simulink model "HybridReactorController"  (R2013a)
settings: Solver=ode45  StartTime=0.0  StopTime=500  RelTol=1e-3
undefined symbols (not defined in the file or in its folder): DiscIntNeverNeededParam
settings Model: Creator=Avisek Naug  LastModifiedBy=Avisek Naug

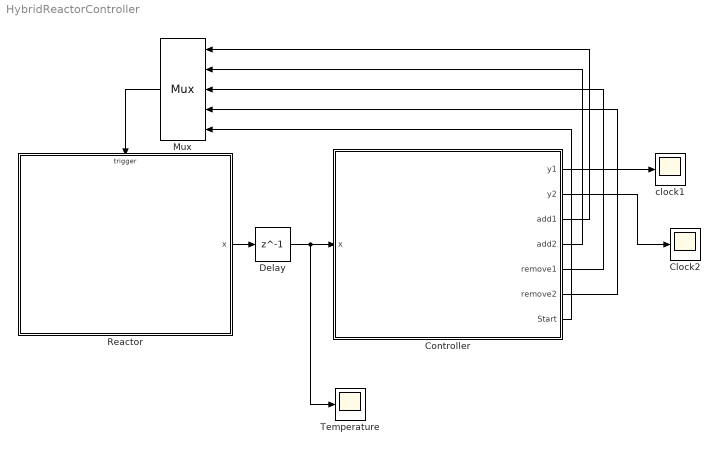
== system HybridReactorController ==
  Clock2 : Scope
      settings: SaveName=ScopeData2
  Controller : Stateflow chart  TreatAsAtomicUnit=on
  Delay : Delay  DelayLength=1  InitialCondition=0  SampleTime=5
  Mux : Mux  Inputs=5
      settings: DisplayOption=signals
  Reactor : Stateflow chart  TreatAsAtomicUnit=on
  Temperature : Scope
  clock1 : Scope
  wires:
  Reactor/1(x) -> Delay/1
  Mux/1 -> Reactor/Trigger
  Controller/3(add1) -> Mux/1
  Controller/4(add2) -> Mux/2
  Controller/5(remove1) -> Mux/3
  Controller/6(remove2) -> Mux/4
  Delay/1 -> Controller/1(x), Temperature/1
  Controller/1(y1) -> clock1/1
  Controller/2(y2) -> Clock2/1
  Controller/7(Start) -> Mux/5

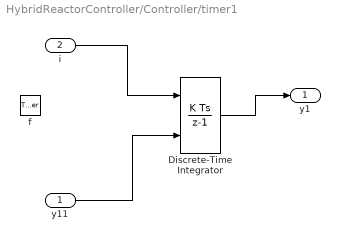
== system HybridReactorController/Controller/timer1 ==
  y11 : Inport  OutDataTypeStr=double
  i : Inport  Port=2
  f : TriggerPort  TriggerType=function-call
      settings: CopyFcn=Stateflow.SLINSF.SimulinkMan.removeBlockPreDeleteFcn  PreDeleteFcn=Stateflow.SLINSF.SimulinkMan.unsafePredeleteFcn
  Discrete-Time Integrator : DiscreteIntegrator  InitialConditionSource=external  SampleTime=-1  ICPrevOutput=DiscIntNeverNeededParam  ICPrevScaledInput=DiscIntNeverNeededParam
  y1 : Outport
  wires:
  Discrete-Time Integrator/1 -> y1/1
  i/1 -> Discrete-Time Integrator/1
  y11/1 -> Discrete-Time Integrator/2

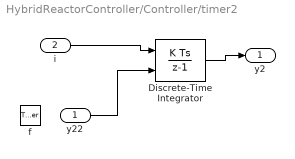
== system HybridReactorController/Controller/timer2 ==
  y22 : Inport
  i : Inport  Port=2
  f : TriggerPort  TriggerType=function-call
      settings: CopyFcn=Stateflow.SLINSF.SimulinkMan.removeBlockPreDeleteFcn  PreDeleteFcn=Stateflow.SLINSF.SimulinkMan.unsafePredeleteFcn
  Discrete-Time Integrator : DiscreteIntegrator  InitialConditionSource=external  SampleTime=-1  ICPrevOutput=DiscIntNeverNeededParam  ICPrevScaledInput=DiscIntNeverNeededParam
  y2 : Outport
  wires:
  Discrete-Time Integrator/1 -> y2/1
  y22/1 -> Discrete-Time Integrator/2
  i/1 -> Discrete-Time Integrator/1

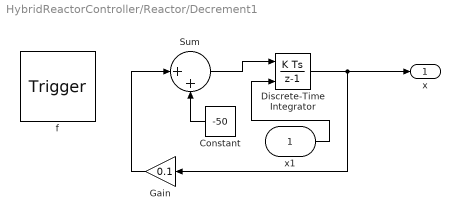
== system HybridReactorController/Reactor/Decrement1 ==
  x1 : Inport
  f : TriggerPort  TriggerType=function-call
      settings: CopyFcn=Stateflow.SLINSF.SimulinkMan.removeBlockPreDeleteFcn  PreDeleteFcn=Stateflow.SLINSF.SimulinkMan.unsafePredeleteFcn
  Constant : Constant  Value=-50
  Discrete-Time Integrator : DiscreteIntegrator  InitialConditionSource=external  SampleTime=-1  ICPrevOutput=DiscIntNeverNeededParam  ICPrevScaledInput=DiscIntNeverNeededParam
  Gain : Gain  Gain=0.1
  Sum : Sum  Inputs=|++
  x : Outport
  wires:
  Sum/1 -> Discrete-Time Integrator/1
  Gain/1 -> Sum/1
  Constant/1 -> Sum/2
  Discrete-Time Integrator/1 -> Gain/1, x/1
  x1/1 -> Discrete-Time Integrator/2

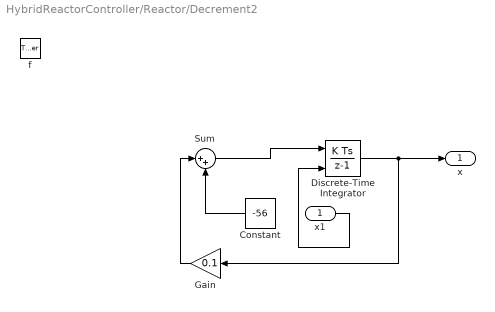
== system HybridReactorController/Reactor/Decrement2 ==
  x1 : Inport
  f : TriggerPort  TriggerType=function-call
      settings: CopyFcn=Stateflow.SLINSF.SimulinkMan.removeBlockPreDeleteFcn  PreDeleteFcn=Stateflow.SLINSF.SimulinkMan.unsafePredeleteFcn
  Constant : Constant  Value=-56
  Discrete-Time Integrator : DiscreteIntegrator  InitialConditionSource=external  SampleTime=-1  ICPrevOutput=DiscIntNeverNeededParam  ICPrevScaledInput=DiscIntNeverNeededParam
  Gain : Gain  Gain=0.1
  Sum : Sum  Inputs=|++
  x : Outport
  wires:
  Sum/1 -> Discrete-Time Integrator/1
  Gain/1 -> Sum/1
  Constant/1 -> Sum/2
  Discrete-Time Integrator/1 -> Gain/1, x/1
  x1/1 -> Discrete-Time Integrator/2

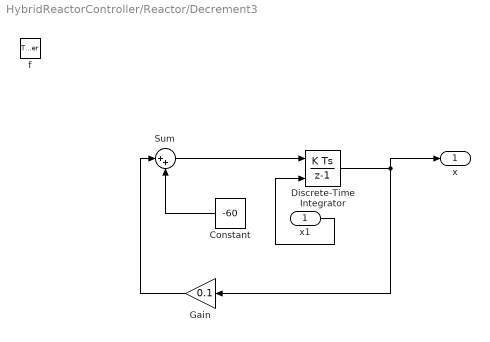
== system HybridReactorController/Reactor/Decrement3 ==
  x1 : Inport
  f : TriggerPort  TriggerType=function-call
      settings: CopyFcn=Stateflow.SLINSF.SimulinkMan.removeBlockPreDeleteFcn  PreDeleteFcn=Stateflow.SLINSF.SimulinkMan.unsafePredeleteFcn
  Constant : Constant  Value=-60
  Discrete-Time Integrator : DiscreteIntegrator  InitialConditionSource=external  SampleTime=-1  ICPrevOutput=DiscIntNeverNeededParam  ICPrevScaledInput=DiscIntNeverNeededParam
  Gain : Gain  Gain=0.1
  Sum : Sum  Inputs=|++
  x : Outport
  wires:
  Discrete-Time Integrator/1 -> x/1, Gain/1
  Gain/1 -> Sum/1
  Constant/1 -> Sum/2
  Sum/1 -> Discrete-Time Integrator/1
  x1/1 -> Discrete-Time Integrator/2

== stateflow chart HybridReactorController/Reactor ==
  state Rod1
    en:
    x1 = x;
    du:
    x = Decrement2(x1);
  state NoRod
    en:
    x1 = x ;
    du:
    x = Decrement1(x1);
  state Rod2
    en:
    x1 = x;
    du:
    x =Decrement3(x1);
  state x = Decrement1(x1) [function]
  state x = Decrement2(x1) [function]
  state x = Decrement3(x1) [function]
  NoRod -> Rod1 [order 1] : add1
  (default) -> NoRod : Start{x= 510;}
  Rod1 -> NoRod : remove1
  NoRod -> Rod2 [order 2] : add2
  Rod2 -> NoRod : remove2
  data: x1 function_input; x function_output; x1 function_input; x function_output; x1 function_input; x function_output; x output double; x1 local double
  events: add1 input EITHER_EDGE_EVENT; add2 input EITHER_EDGE_EVENT; remove1 input EITHER_EDGE_EVENT; remove2 input EITHER_EDGE_EVENT; Start input EITHER_EDGE_EVENT

== stateflow chart HybridReactorController/Controller ==
  state Rod1
    en:
    y11 = y1;
    y22 = y2;
    i = 1;
    du:
    y1 = timer1(y11,i);
    y2 = timer2(y22,i);
  state y1 = timer1(y11,i) [function]
  state NoRod
    en:
    y11 = y1;
    y22 = y2;
    i = 1;
    du:
    y1 = timer1(y11,i);
    y2 = timer2(y22,i);
  state Rod2
    en:
    y11 = y1;
    y22 = y2;
    i = 1;
    du:
    y1 = timer1(y11,i);
    y2 = timer2(y22,i);
  state y2 = timer2(y22,i) [function]
  NoRod -> Rod1 [order 1] : [x>=510&y1>=50&y2<50]/{send(add1)}
  (default) -> NoRod : {y1 = 50;
      | y2 = 50;send(Start);}
  Rod1 -> NoRod : [x<=510]/{send(remove1);y1=0;}
  NoRod -> Rod2 [order 2] : [x>=550&y2>=50]/{send(add2)}
  Rod2 -> NoRod : [x<=510]/{send(remove2);y2=0;}
  data: y1 function_output; y11 function_input double; i function_input; y22 function_input; y2 function_output; i function_input; x input double; y1 output double; y2 output double; i local double; y11 local double; y22 local double
  events: add1 output EITHER_EDGE_EVENT; add2 output EITHER_EDGE_EVENT; remove1 output EITHER_EDGE_EVENT; remove2 output EITHER_EDGE_EVENT; Start output EITHER_EDGE_EVENT
